simulink model "SalirClaseWaypoints"  (R2022b)
settings: Solver=FixedStepAuto  StartTime=0.0  StopTime=100  RelTol=1e-3  EnableMultiTasking=on
libraries: slpidlib x1, robotalgslib x1
settings Model: ExtModeTrigDuration=2  Creator=Usuario_UMA  LastModifiedBy=Usuario
settings OptimizationCC: EnhancedBackFolding=on  PassReuseOutputArgsAs=Individual arguments  ZeroExternalMemoryAtStartup=off  ZeroInternalMemoryAtStartup=off  MaxStackSize=64  OptimizeBlockOrder=speed  DifferentSizesBufferReuse=on  EfficientTunableParamExpr=on
settings DebuggingCC: ParameterTunabilityLossMsg=error
settings HardwareCC: ProdBitPerInt=16  ProdBitPerPointer=16  ProdBitPerSizeT=16  ProdBitPerPtrDiffT=16  ProdLargestAtomicFloat=None  ProdWordSize=8  ProdHWDeviceType=Atmel->AVR  UseEmbeddedCoderFeatures=off
settings SFSimCC: MATLABDynamicMemAlloc=off
settings RTWCC: Description=Embedded Coder  SystemTargetFile=ert.tlc  HardwareBoard=Arduino Mega 2560  TLCOptions=-aInlineSetEventsForThisBaseRateFcn=TLC_FALSE -aSuppressMultiTaskScheduler=TLC_FALSE -aRateBasedStepFcn=1  TemplateMakefile=ert_default_tmf  Toolchain=Arduino AVR  BuildConfiguration=Faster Runs
settings CodeAppCC: ForceParamTrailComments=on  IgnoreCustomStorageClasses=off  OperatorAnnotations=on  SimulinkDataObjDesc=on  SFDataObjDesc=on  InsertBlockDesc=on
settings ERTTargetCC: SupportContinuousTime=on  SupportNonInlinedSFcns=on  SupportVariableSizeSignals=on  ExtModeTransport=3  ExtModeStaticAlloc=on  ExtModeAutomaticAllocSize=off  ExtModeStaticAllocSize=2048  ExtModeMexFile=ext_xcp  ExtModeIntrfLevel=Level2 - Open

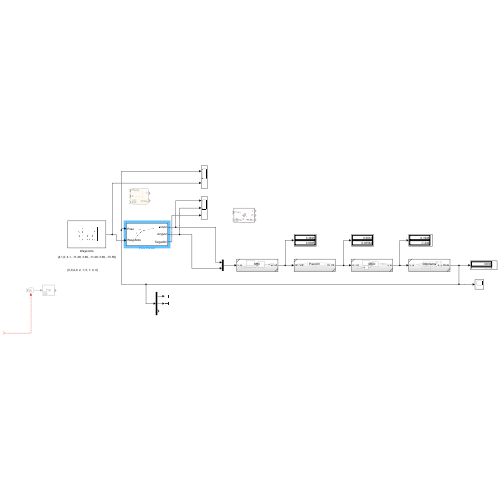
[thumbnail: Simulink's stored preview of the top-level diagram]
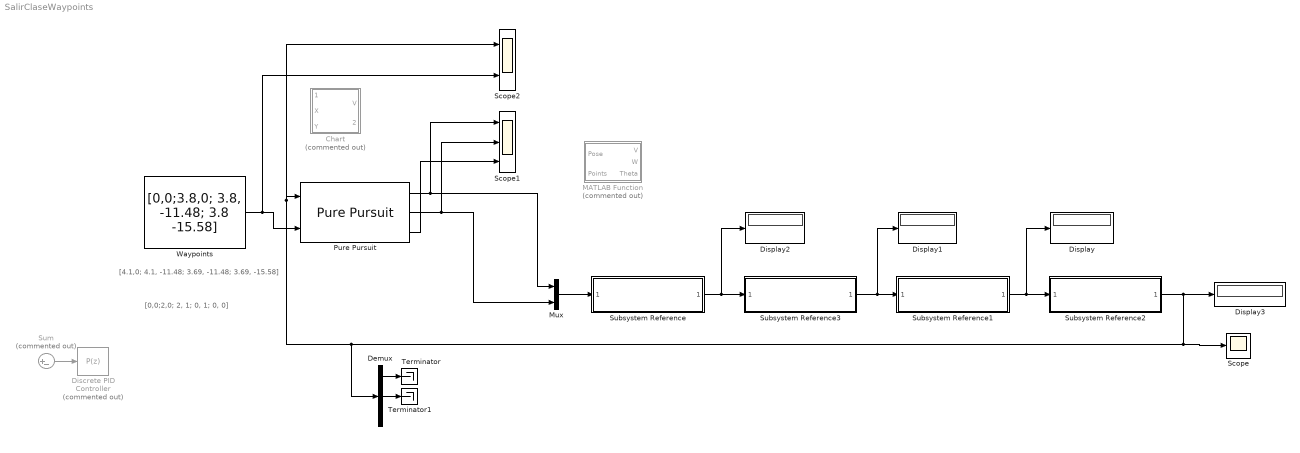
== system SalirClaseWaypoints ==
  note: [0,0;2,0; 2, 1; 0, 1; 0, 0]
  note: [4.1,0; 4.1, -11.48; 3.69, -11.48; 3.69, -15.58]
  Chart : Stateflow chart  Commented=on  TreatAsAtomicUnit=on
  Demux : Demux  Outputs=3
  Discrete PID Controller : slpidlib/PID Controller  Commented=on  Controller=P  Form=Parallel  TimeDomain=Discrete-time  UseExternalTs=off  SampleTime=-1  IntegratorMethod=Forward Euler  FilterMethod=Forward Euler  ControllerParametersSource=internal  P=1  I=1  UseKiTs=off  D=0  N=100  UseFilter=on  TunerSelectOption=Transfer Function Based (PID Tuner App)  InitialConditionSource=internal  InitialConditionForIntegrator=0  InitialConditionForFilter=0  DifferentiatorICPrevScaledInput=0  ExternalReset=none  TrackingMode=off  Kt=1  LimitOutput=off  SatLimitsSource=internal  UpperSaturationLimit=inf  LowerSaturationLimit=-inf  LinearizeAsGain=off  AntiWindupMode=none  Kb=1  LimitIntegrator=off  UpperIntegratorSaturationLimit=inf  LowerIntegratorSaturationLimit=-inf  POutMin=[]  POutMax=[]  IOutMin=[]  IOutMax=[]  DOutMin=[]  DOutMax=[]  NOutMin=[]  NOutMax=[]  SumOutMin=[]  SumOutMax=[]  SaturationOutMin=[]  SaturationOutMax=[]  PParamMin=[]  PParamMax=[]  IParamMin=[]  IParamMax=[]  DParamMin=[]  DParamMax=[]  NParamMin=[]  NParamMax=[]  KbParamMin=[]  KbParamMax=[]  KtParamMin=[]  KtParamMax=[]  KbOutMin=[]  KbOutMax=[]  KtOutMin=[]  KtOutMax=[]  IntegratorOutMin=[]  IntegratorOutMax=[]  FilterOutMin=[]  FilterOutMax=[]  SumI1OutMin=[]  SumI1OutMax=[]  SumI2OutMin=[]  SumI2OutMax=[]  SumI3OutMin=[]  SumI3OutMax=[]  SumI4OutMin=[]  SumI4OutMax=[]  SumDOutMin=[]  SumDOutMax=[]  DifferentiatorOutMin=[]  DifferentiatorOutMax=[]  FilterDiffOutCoefMin=[]  FilterDiffOutCoefMax=[]  ReciprocalOutMin=[]  ReciprocalOutMax=[]  SumDenOutMin=[]  SumDenOutMax=[]  SumNumOutMin=[]  SumNumOutMax=[]  DivideOutMin=[]  DivideOutMax=[]  UdiffTsProdOutMin=[]  UdiffTsProdOutMax=[]  NTsProdOutMin=[]  NTsProdOutMax=[]  UintegralTsProdOutMin=[]  UintegralTsProdOutMax=[]  UngainTsProdOutMin=[]  UngainTsProdOutMax=[]  ClampingZeroOutDataTypeStr=Inherit: Inherit via back propagation  ClampingZeroOutMin=[]  ClampingZeroOutMax=[]  FilterDenConstantOutDataTypeStr=Inherit: Inherit via back propagation  FilterDenConstantOutMin=[]  FilterDenConstantOutMax=[]  PCopyOutDataTypeStr=Inherit: Inherit via back propagation  PCopyOutMin=[]  PCopyOutMax=[]  NCopyOutDataTypeStr=Inherit: Inherit via back propagation  NCopyOutMin=[]  NCopyOutMax=[]  IntegratorContinuousStateAttributes=''  IntegratorStateMustResolveToSignalObject=off  IntegratorRTWStateStorageClass=Auto  FilterContinuousStateAttributes=''  FilterStateMustResolveToSignalObject=off  FilterRTWStateStorageClass=Auto  ParallelPVariant=InternalParameters  IdealPVariant=Disabled  IVariant=Disabled  DVariant=Disabled  IntegratorVariant=Disabled  SatVariant=Disabled  AWVariant=Disabled  PCopyVariant=Disabled  TRVariant=Disabled  FdbkBlocksVariant=Forward  IdealPFdbkVariant=Disabled  SatFdbkVariant=Disabled  DerivativeFilterVariant=Disabled  NVariant=Disabled  NCopyVariant=Disabled_SignalSpec  FilterICVariant=Disabled  IntegratorICVariant=Disabled  ExternalResetVariant=Disabled  TRSumVariant=Passthrough  SumFdbkVariant=Disabled  SumVariant=Passthrough_P  TsampFilterVariant=InternalTs  TsampNgainVariant=Passthrough  TsampIntegralVariant=Disabled_SignalSpec  ExternalSaturationOutDataTypeStr=Inherit: Same as second input
      settings: LibrarySourceBlock=simulink/Discrete/Discrete PID Controller
  Display{,1..3} (4 alike) : Display
  MATLAB Function : MATLAB Function  Commented=on  TreatAsAtomicUnit=on
  Mux : Mux  Inputs=2
  Pure Pursuit : robotalgslib/Pure Pursuit  DesiredLinearVelocity=0.2  MaxAngularVelocity=1.5  LookaheadDistance=0.2  TargetDirPort=on  SimulateUsing=Code generation
      settings: LibrarySourceBlock=navlib/Control Algorithms/Pure Pursuit
  Scope : Scope
  Scope1 : Scope  NumInputPorts=3
  Scope2 : Scope  NumInputPorts=2
  Subsystem Reference : Subsystem  ReferencedSubsystem=MCI
  Subsystem Reference1 : Subsystem  ReferencedSubsystem=MCD
  Subsystem Reference2 : Subsystem  ReferencedSubsystem=Odometria
  Subsystem Reference3 : Subsystem  ReferencedSubsystem=PieroCV
  Sum : Sum  Commented=on  Inputs=|+-
  Terminator : Terminator
  Terminator1 : Terminator
  Waypoints : Constant  Value=[0,0;3.8,0; 3.8, -11.48; 3.8 -15.58]
  wires:
  Pure Pursuit/2 -> Scope1/2, Mux/2
  Subsystem Reference3/1 -> Display1/1, Subsystem Reference1/1
  Demux/2 -> Terminator1/1
  Subsystem Reference2/1 -> Scope/1, Scope2/1, Pure Pursuit/1, Demux/1, Display3/1
  Demux/1 -> Terminator/1
  Subsystem Reference1/1 -> Display/1, Subsystem Reference2/1
  Mux/1 -> Subsystem Reference/1
  Subsystem Reference/1 -> Display2/1, Subsystem Reference3/1
  Pure Pursuit/1 -> Scope1/1, Mux/1
  Waypoints/1 -> Scope2/2, Pure Pursuit/2
  ? -> Sum/2
  Sum/1 -> Discrete PID Controller/1
  Pure Pursuit/3 -> Scope1/3

== matlab function SalirClaseWaypoints/MATLAB Function ==
  data: Pose input; V output; Points input; W output; Theta output
function [V, W, Theta] = PurePursuit(Pose, Points)
x = Points(:,1)';
y = Points(:,2)';

robot_x = Pose(1);
robot_y = Pose(2);
robot_theta = Pose(3);

n = length(x);

lookahead = 0.2;    %umbral de cambio al siguiente punto
linear_vel = 0.205; w_max = 1.5;

persistent index;
if isempty(index)
    index = 1;
end

if (index < n)
    target_x = x(index);
    target_y = y(index);
    
    % Distancia y ángulo al punto objetivo
    distance = sqrt((target_x - robot_x)^2 + (target_y - robot_y)^2);
    angle = atan2(target_y - robot_y, target_x - robot_x) - robot_theta;
    
    if distance < lookahead     % Cambiar por un while
        index = index +1;
    end

    Theta = angle;
    V = linear_vel;

    if (lookahead < 1.0)
        R = ((lookahead+0.1)/(2*sin(angle)));
    else
        R = (lookahead/(2*sin(angle)));
    end

    W = 0.25 / R;

    if (W > w_max)
        W = w_max;
    end
else
    W = 0;  V = 0;

end

end

== stateflow chart SalirClaseWaypoints/Chart ==
  state Paro
    V=0;
    Theta=0;
  state Tramo10A
    entry:
    V=0.205;
    Theta=0;
  state GiroDer1
    entry:
    V=0.05;
    Theta=-pi/2;
  state Tramo28A
    entry:
    V=0.205;
    Theta=-pi/2;
  state GiroDer3
    entry:
    V=0.05;
    Theta=-pi/2;
  state Tramo1A
    entry:
    V=0.205;
    Theta=0;
  state GiroDer2
    entry:
    V=0.05;
    Theta=-pi;
  state Tramo10A2
    entry:
    V=0.205;
    Theta=-pi/2;
  state FIN
    entry:
    V=0;
    Theta=-pi/2;
  (default) -> Paro
  Paro -> Tramo10A : after(2,sec)
  Tramo10A -> GiroDer1 : [X>=4.1]
  GiroDer1 -> Tramo28A : [iTheta<=(-pi/2)]
  Tramo28A -> GiroDer2 : [Y<=-11.48]
  Tramo1A -> GiroDer3 : [X<=3.69]
  GiroDer2 -> Tramo1A : [iTheta<=-pi]
  GiroDer3 -> Tramo10A2 : [iTheta>=(-pi/2)]
  Tramo10A2 -> FIN : [Y<=-15.58]
  data: iTheta input; X input; Y input; V output; Theta output
